simulink model "Question3"  (R2020a)
settings: Solver=FixedStepAuto  StartTime=0.0  StopTime=10.0  FixedStep=0.001  RelTol=1e-3
settings Model: Creator=aishw  LastModifiedBy=aishw

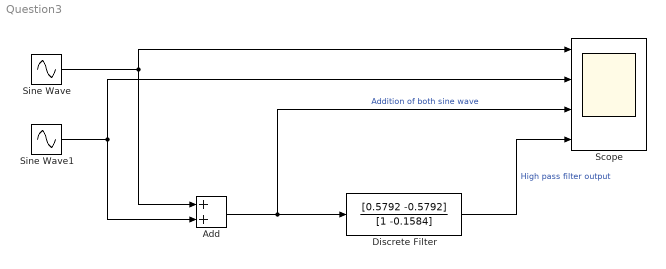
== system Question3 ==
  Add : Sum
  Discrete Filter : DiscreteFilter  Numerator=[0.5792 -0.5792]  Denominator=[1 -0.1584]
  Scope : Scope  NumInputPorts=4
  Sine Wave : Sin  Amplitude=50  SampleTime=0
  Sine Wave1 : Sin  Amplitude=5  Frequency=10  SampleTime=0
  wires:
  Sine Wave/1 -> Add/1, Scope/1
  Add/1 -> Scope/3, Discrete Filter/1  "Addition of both sine wave"
  Sine Wave1/1 -> Add/2, Scope/2
  Discrete Filter/1 -> Scope/4  "High pass filter output"
